simulink model "Figure_3_1_TP_Telecom_modulation_QUAM64"  (R2020a)
settings: Solver=VariableStepAuto  StartTime=0.0  StopTime=2000/9e6  RelTol=1e-3
libraries: commrandsrc3 x1, commdigbbndam3 x1, dspsrcs4 x1
settings Model: Creator=iba  LastModifiedBy=iba

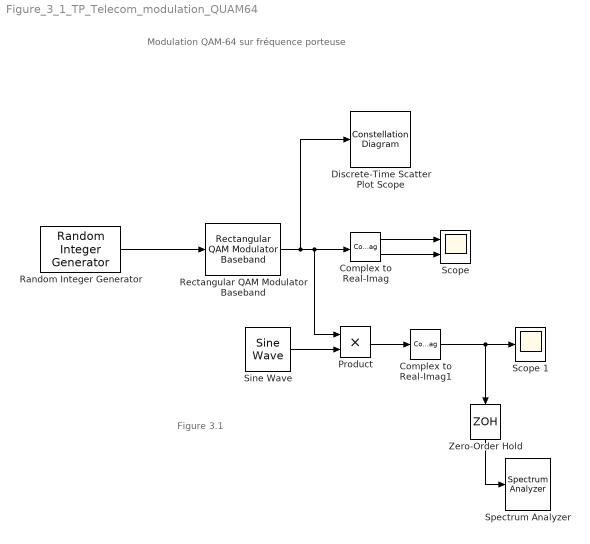
== system Figure_3_1_TP_Telecom_modulation_QUAM64 ==
  note: Figure 3.1
  note: Modulation QAM-64 sur fréquence porteuse
  Complex to Real-Imag : ComplexToRealImag
  Complex to Real-Imag1 : ComplexToRealImag  Output=Real
  Discrete-Time Scatter Plot Scope : ConstellationDiagram
  Product : Product
  "Random Integer Generator " : commrandsrc3/Random Integer Generator  SetSize=64  SeedSource=Parameter  Seed=37  SampleTime=1/9e6  SamplesPerFrame=1  OutputDataType=double  SimulateUsing=Interpreted execution
  Rectangular QAM Modulator Baseband : commdigbbndam3/Rectangular QAM Modulator Baseband  M=64  InType=Integer  Enc=Gray  Mapping=[0:15]  PowType=Min. distance between symbols  MinDist=2  AvgPow=1  PeakPow=1  Ph=0  outDtype=double  outWordLen=16  outUDDataType=sfix(16)  outFracLenMode=Best precision  outFracLen=15  outDataTypeStr=double  outLastDataTypeStr=double
  "Scope " : Scope  NumInputPorts=2
  Scope 1 : Scope
  Sine Wave : dspsrcs4/Sine Wave  Amplitude=1  Frequency=9e6  Phase=0  SampleMode=Discrete  OutComplex=Complex  CompMethod=Trigonometric fcn  TableSize=Speed  SampleTime=1/10.5e9  SamplesPerFrame=1  ResetState=Restart at time zero  OutputFrames=off  dataType=double  wordLen=16  udDataType=sfix(16)  fracBitsMode=Best precision  numFracBits=15  OutDataTypeStr=double  LastOutDataTypeStr=double
  "Spectrum Analyzer " : SpectrumAnalyzer
  Zero-Order Hold : ZeroOrderHold  SampleTime=1/54e6
  wires:
  "Random Integer Generator "/1 -> Rectangular QAM Modulator Baseband/1
  Sine Wave/1 -> Product/2
  Complex to Real-Imag/1 -> "Scope "/1
  Complex to Real-Imag/2 -> "Scope "/2
  Product/1 -> Complex to Real-Imag1/1
  Complex to Real-Imag1/1 -> Zero-Order Hold/1, Scope 1/1
  Zero-Order Hold/1 -> "Spectrum Analyzer "/1
  Rectangular QAM Modulator Baseband/1 -> Complex to Real-Imag/1, Product/1, Discrete-Time Scatter Plot Scope/1
